simulink model "BotModel2Sens"  (R2025a)
settings: Solver=VariableStepAuto  StartTime=0.0  StopTime=2  FixedStep=0.01  RelTol=1e-3
values from neighbouring files (symbols this model uses):
  Achsabstand = 0.15    [Model1Sensibilities.m]    (also in Model1numericalPSA.m; Model2Sensibilities.m; Modellvalidierung.m; MotorSens2.m)
  B_dis = 0.25    [Model1Sensibilities.m]    (also in Model1numericalPSA.m = 0.15; Model2Sensibilities.m; Modellvalidierung.m = 0.15; MotorSens2.m)
  c_pose = [0 0 0 0 1 0 0 ... (first row only)    [Model2Sensibilities.m]    (also in ParamsModell.m; ParamsModell2.m; model1Sensibiliaet.m; robotmodel2Sensibilities.m)
  g = 9.81    [Model1Sensibilities.m]    (also in Model1numericalPSA.m; Model2Sensibilities.m; Modellvalidierung.m; MotorSens2.m)
  I_Bot = 0.0072    [Model1Sensibilities.m]    (also in Model1numericalPSA.m; Model2Sensibilities.m; Modellvalidierung.m; MotorSens2.m)
  I_Reifen = 1.8 * 10^-5    (= 1.8e-05)    [Model1Sensibilities.m]    (also in Model1numericalPSA.m; Model2Sensibilities.m; Modellvalidierung.m; ParamsModell.m)
  L_B = 0.12    [Model1numericalPSA.m]    (also in Modellvalidierung.m; ParamsModell.m; model1Sensibiliaet.m; robotmodel1Sensibilities.m)
  m_ges = 1    [Model1Sensibilities.m]    (also in Model1numericalPSA.m; Model2Sensibilities.m; Modellvalidierung.m; MotorSens2.m)
  motor_BackEMFkoef = 0.0035    [Model1Sensibilities.m]    (also in Model1numericalPSA.m; Model2Sensibilities.m; Modellvalidierung.m; MotorSens2.m)
  motor_Daempfung = 9.12 * 10^-8    (= 9.12e-08)    [Model1Sensibilities.m]    (also in Model1numericalPSA.m; Model2Sensibilities.m; Modellvalidierung.m; MotorSens2.m)
  motor_Drehmomentkoef = 0.0174    [Model1Sensibilities.m]    (also in Model1numericalPSA.m = 0.0035; Model2Sensibilities.m; Modellvalidierung.m = 0.0035; MotorSens2.m)
  motor_Induktivitaet = 0.0002    [Model1Sensibilities.m]    (also in Model1numericalPSA.m; Model2Sensibilities.m; Modellvalidierung.m; MotorSens2.m)
  motor_traegheit = 0.847 * 10^-6    (= 8.47e-07)    [Model1Sensibilities.m]    (also in Model1numericalPSA.m; Model2Sensibilities.m; Modellvalidierung.m; MotorSens2.m)
  motor_Widerstand = 13.33    [Model1Sensibilities.m]    (also in Model1numericalPSA.m; Model2Sensibilities.m; Modellvalidierung.m; MotorSens2.m)
  Motoruebersetzung = 100    [Model1Sensibilities.m]    (also in Model1numericalPSA.m; Model2Sensibilities.m; Modellvalidierung.m; MotorSens2.m)
  mue_g = 0.1    [Model1Sensibilities.m]    (also in Model1numericalPSA.m; Model2Sensibilities.m; Modellvalidierung.m; MotorSens2.m)
  Reifen_Radius = 0.04    [Model1Sensibilities.m]    (also in Model1numericalPSA.m; Model2Sensibilities.m; Modellvalidierung.m; MotorSens2.m)
  x0s = [0 ... (first row only)    [Model2Sensibilities.m]    (also in MotorSens2.m = [; Motor_Sensitivitaet.m = [; Parameter.m = [; ParamsModell.m)
  Xi = 2/3    (= 0.666666666667)    [Model1Sensibilities.m]    (also in Model1numericalPSA.m = 0.333333333333; Model2Sensibilities.m; Modellvalidierung.m = 0.333333333333; MotorSens2.m)
settings Model: Creator=jakob  LastModifiedBy=jakob

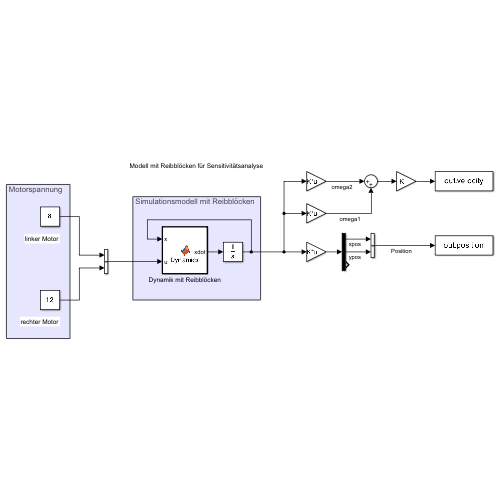
[thumbnail: Simulink's stored preview of the top-level diagram]
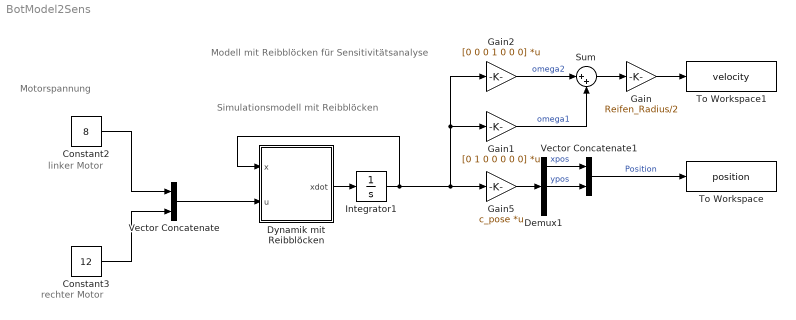
== system BotModel2Sens ==
  note: Simulationsmodell mit Reibblöcken
  note: Modell mit Reibblöcken für Sensitivitätsanalyse
  note: rechter Motor
  note: linker Motor
  note: Motorspannung
  Constant2 : Constant  Value=8  SampleTime=1
  Constant3 : Constant  Value=12  SampleTime=1
  Demux1 : Demux  Outputs=3
  Dynamik mit Reibblöcken : MATLAB Function  TreatAsAtomicUnit=on
  Gain : Gain  Gain=Reifen_Radius/2
  Gain1 : Gain  Gain=[0 1 0 0 0 0 0]  Multiplication=Matrix(K*u)
  Gain2 : Gain  Gain=[0 0 0 1 0 0 0]  Multiplication=Matrix(K*u)
  Gain5 : Gain  Gain=c_pose  Multiplication=Matrix(K*u)
  Integrator1 : Integrator  InitialCondition=x0s
  Sum : Sum  Inputs=|++
  To Workspace : ToWorkspace  VariableName=position  SaveFormat=Timeseries  SampleTime=-1
  To Workspace1 : ToWorkspace  VariableName=velocity  SaveFormat=Timeseries  SampleTime=-1
  Vector Concatenate : Concatenate
  Vector Concatenate1 : Concatenate
  wires:
  Sum/1 -> Gain/1
  Vector Concatenate/1 -> Dynamik mit Reibblöcken/2(u)
  Gain1/1 -> Sum/2  "omega1"
  Integrator1/1 -> Dynamik mit Reibblöcken/1(x), Gain2/1, Gain1/1, Gain5/1
  Gain2/1 -> Sum/1  "omega2"
  Gain/1 -> To Workspace1/1
  Dynamik mit Reibblöcken/1(xdot) -> Integrator1/1
  Gain5/1 -> Demux1/1
  Constant2/1 -> Vector Concatenate/1
  Constant3/1 -> Vector Concatenate/2
  Demux1/1 -> Vector Concatenate1/1  "xpos"
  Demux1/2 -> Vector Concatenate1/2  "ypos"
  Vector Concatenate1/1 -> To Workspace/1  "Position"

== matlab function BotModel2Sens/Dynamik mit Reibblöcken ==
  data: x input; u input; xdot output; Motoruebersetzung parameter; motor_traegheit parameter; m_ges parameter; Reifen_Radius parameter; I_Bot parameter; Achsabstand parameter; motor_Drehmomentkoef parameter; motor_Daempfung parameter; motor_Widerstand parameter; motor_Induktivitaet parameter; motor_BackEMFkoef parameter; mue_g parameter; g parameter; Xi parameter; B_dis parameter; I_Reifen parameter; L_B parameter
function xdot = Dynamics(x,u,Motoruebersetzung, motor_traegheit, m_ges, Reifen_Radius, I_Bot, Achsabstand, motor_Drehmomentkoef, motor_Daempfung,motor_Widerstand, motor_Induktivitaet, motor_BackEMFkoef,mue_g, g, Xi, B_dis,I_Reifen,L_B)

%% Input
%x-vec:
i_m1 = x(1);
om_m1 = x(2);
i_m2 = x(3);
om_m2 = x(4);
theta = x(7);

%Spannungs-Eingang
Ue1 = u(1);
Ue2 = u(2);

%% Träheitstensor
J_Mn = Motoruebersetzung^2 * motor_traegheit;
C1 = (m_ges*Reifen_Radius^2)/4 - (I_Bot*Reifen_Radius^2)/(Achsabstand^2);
C2 = (m_ges*Reifen_Radius^2)/4 + (I_Bot*Reifen_Radius^2)/(Achsabstand^2);

M11 = J_Mn + C1 + I_Reifen;
M12 = C2;
M21 = M12;
M22 = M11;

J_g = [M11 M12;
       M21 M22];


%% Berechnung der Belastungen
% Grenzgeschwindigkeit gegen 0
v_Tresh = 1e-3;
% Grenzwinkelgeschwindigkeit gegen 0
omega_Tresh = 1e-3;
% Grenzwinkelgeschwindigkeits-Unterschied
eps_om = 1e-6;
% Steigungen für Glättungsfunktionen
k_smooth = 5000;
k_xppos = 100;
k_xp = 5 / eps_om;
% konstante Nenner-Erwiterungen für Singlaritäten
delta_sig_sq = 1e-6;
xp_delta = 1e-6;
eta_abs_sq = (eps_om/10)^2;

% Angriffspunkte der Reibngskräfte
B1 = [(1-Xi)*B_dis; L_B/2];
B2 = [(1-Xi)*B_dis; -L_B/2];

% Berechnung der reibungskraft-Angriffswinkel über Ermittlung von
% Geschwindigkeitspol xp
OmegaSum = om_m1 + om_m2;
deltaOmega = om_m2-om_m1;
smooth_abs_DeltaOmega = sqrt(deltaOmega^2 + eta_abs_sq);

v_Bot = (Reifen_Radius/2)*OmegaSum;
omega_Bot = (Reifen_Radius/Achsabstand)*smooth_abs_DeltaOmega;

% Glättungsfunktionen für Reibungskraft-> keine Reibung bei v_Bot / omega_Bot =0
smooth_factor_straight = 0.5 * (1 + tanh(k_smooth * (v_Bot - v_Tresh)));
smooth_factor_spin = 0.5 * (1 + tanh(k_smooth * (omega_Bot - omega_Tresh)));
C_Frb = mue_g * m_ges * g * (Xi/2);
Frb_smooth_straight = smooth_factor_straight * C_Frb;
Frb_smooth_spin = smooth_factor_spin * C_Frb;

% Bestimmung von Geschwndigkeitspol xp
w = 0.5 * (1 + tanh(k_xp*(smooth_abs_DeltaOmega - eps_om)));

inv_xp_A_const = 1e-6;

inv_xp_B_turn_nun = (2/Achsabstand) * deltaOmega * OmegaSum;
inv_xp_B_turn_dun = OmegaSum^2 + delta_sig_sq;
inv_xp_B_turn = inv_xp_B_turn_nun / inv_xp_B_turn_dun;

inv_xp_smooth = (1-w) * inv_xp_A_const + w * inv_xp_B_turn;
xp_smooth = 1./(inv_xp_smooth+xp_delta);

xppos_translation = [-Xi*B_dis; xp_smooth];
xppos_turnonpint = [-Xi*B_dis; 0];

s = 1- tanh((k_xppos * OmegaSum)^2);
xppos = (1-s)* xppos_translation + s * xppos_turnonpint;

% Bestimmung von angriffswinkel von Reibkräften
B1xp = xppos - B1;
B2xp = xppos - B2;
Fb1_dir = [B1xp(2);-B1xp(1)];
Fb2_dir = [B2xp(2);-B2xp(1)];
Fb1_dir_unit = Fb1_dir / norm(Fb1_dir);
Fb2_dir_unit = Fb2_dir / norm(Fb2_dir);
FRB1spin = Frb_smooth_spin * Fb1_dir_unit;
FRB2spin = Frb_smooth_spin * Fb2_dir_unit;

% Durch reibungskräfte resultierende Momente am Roboter
M_FR1v = cross([B1;0],[FRB1spin;0]);
M_FR1 = M_FR1v(3);
M_FR2v = cross([B2;0],[FRB2spin;0]);
M_FR2 = M_FR2v(3);

% Gesamte Momenten-Belastung aufgrund der reibung bei Kontaktpunkten
Tr1_smooth = -(Frb_smooth_straight* Reifen_Radius/2) * (Fb1_dir_unit(1) + Fb2_dir_unit(1)) + w*(Reifen_Radius/Achsabstand)*(M_FR1+M_FR2);
Tr2_smooth = -(Frb_smooth_straight* Reifen_Radius/2) * (Fb1_dir_unit(1) + Fb2_dir_unit(1)) - w*(Reifen_Radius/Achsabstand)*(M_FR1+M_FR2);

% Gesamte Belastungen an den Motoren
M_belastungen = [Motoruebersetzung * motor_Drehmomentkoef * i_m1 - Motoruebersetzung^2 * motor_Daempfung*om_m1 + Tr1_smooth;
                 Motoruebersetzung * motor_Drehmomentkoef * i_m2 - Motoruebersetzung^2 * motor_Daempfung*om_m2 + Tr2_smooth];

% Bestimmung von Winkelbeschleunigungen der Motoren
om_dot = J_g \ M_belastungen;

%% Berechnung der Kinematik

%Geschwindigkeit vom Achsenmitelpunkt im inertialfestem Koordinatensystem
V_M_0 = [(Reifen_Radius/2) * (om_m1 + om_m2)*cos(theta);
        (Reifen_Radius/2) * (om_m1 + om_m2)*sin(theta)];

%Winkelgeschwindigkeit des Roboters in der Ebene
Om_Bot = (Reifen_Radius/Achsabstand) * (om_m2-om_m1);

%Rotationsmatrix vom Roboter- ins inertialfeste- Koordinatensystem
A_0B = [cos(theta) -sin(theta);
        sin(theta) cos(theta)];

%Schwerpunktgeschwindigkeit aufgrund der drehung im
%Roboter-Koordinatensystem
Vs_rot_B = [0; B_dis*Xi*Om_Bot]; 

%Gesamt-Schwerpunktgeschwindigkeit des Roboters im inertialfesten
%Koordinatensystem
V_Bots_0 = V_M_0 + A_0B*Vs_rot_B;

%% Aufstellen von x-dot
di1dt = -(motor_Widerstand/motor_Induktivitaet) * i_m1 - (Motoruebersetzung * motor_BackEMFkoef/motor_Induktivitaet) * om_m1 + (1/motor_Induktivitaet)* Ue1;
dom1dt = om_dot(1);
di2dt = -(motor_Widerstand/motor_Induktivitaet) * i_m2 - (Motoruebersetzung * motor_BackEMFkoef/motor_Induktivitaet) * om_m2 + (1/motor_Induktivitaet)* Ue2;
dom2dt = om_dot(2);
vx = V_Bots_0(1);
vy = V_Bots_0(2);
dthetadt = Om_Bot;

xdot = [di1dt;dom1dt;di2dt;dom2dt;vx;vy;dthetadt];
